simulink model "small_office"  (Simulink 8.1)
settings: Solver=FixedStepDiscrete  StartTime=0  StopTime=86400  FixedStep=60  RelTol=1e-3
undefined symbols (not defined in the file or in its folder): OHare, USA_IL_Chicago
libraries: CampusEnergyModeling x1
settings Model: Creator=mwetter  LastModifiedBy=sfrank1  ExtModeAutoUpdateStatusClock=off
settings OptimizationCC: InitFltsAndDblsToZero=on
settings DebuggingCC: SaveWithParameterizedLinksMsg=none
settings SFSimCC: SFSimEnableDebug=off  SFSimOverflowDetection=off  SFSimEcho=off  SimCtrlC=off  SimIntegrity=off  SimParseCustomCode=off
settings RTWCC: GenerateMakefile=off
settings GRTTargetCC: TargetFcnLib=ansi_tfl_tmw.mat

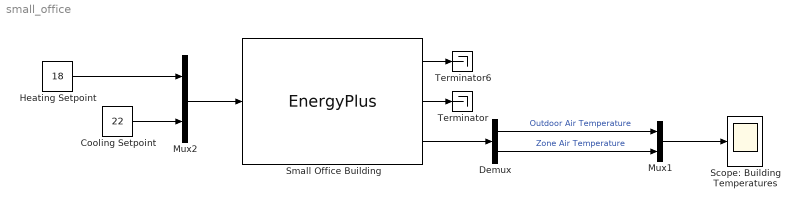
== system small_office ==
  Cooling Setpoint : Constant  Value=22
  Demux : Demux  Outputs=2
  Heating Setpoint : Constant  Value=18
  Mux1 : Mux  Inputs=2
  Mux2 : Mux  Inputs=2
  Scope: Building Temperatures : Scope
      settings: ShowLegends=on  TimeRange=90000  YMin=12  YMax=26
  Small Office Building : CampusEnergyModeling/Buildings/EnergyPlus  work_dir=small_office  rel_path=on  fname=small_office.idf  weather_profile=USA_IL_Chicago-OHare.Intl.AP.725300_TMY3  time_step=60  nout=2  timeout=10  mlep_defaults=on  port=0
  Terminator : Terminator
  Terminator6 : Terminator
  wires:
  Small Office Building/3 -> Demux/1
  Mux2/1 -> Small Office Building/1
  Small Office Building/2 -> Terminator/1
  Small Office Building/1 -> Terminator6/1
  Mux1/1 -> Scope: Building Temperatures/1
  Demux/1 -> Mux1/1  "Outdoor Air Temperature"
  Demux/2 -> Mux1/2  "Zone Air Temperature"
  Heating Setpoint/1 -> Mux2/1
  Cooling Setpoint/1 -> Mux2/2
